simulink model "Kalman_EMPhase_noC"  (R2019b)
settings: Solver=FixedStepAuto  StartTime=0.0  StopTime=model.sim_dur  FixedStep=model.Ts  RelTol=1e-3
undefined symbols (not defined in the file or in its folder): Discrete, model, Time
libraries: dspsrcs4 x10, dspindex x4, ctrlSharedLib x2
settings Model: Creator=isidoraradenkovic  LastModifiedBy=isidoraradenkovic

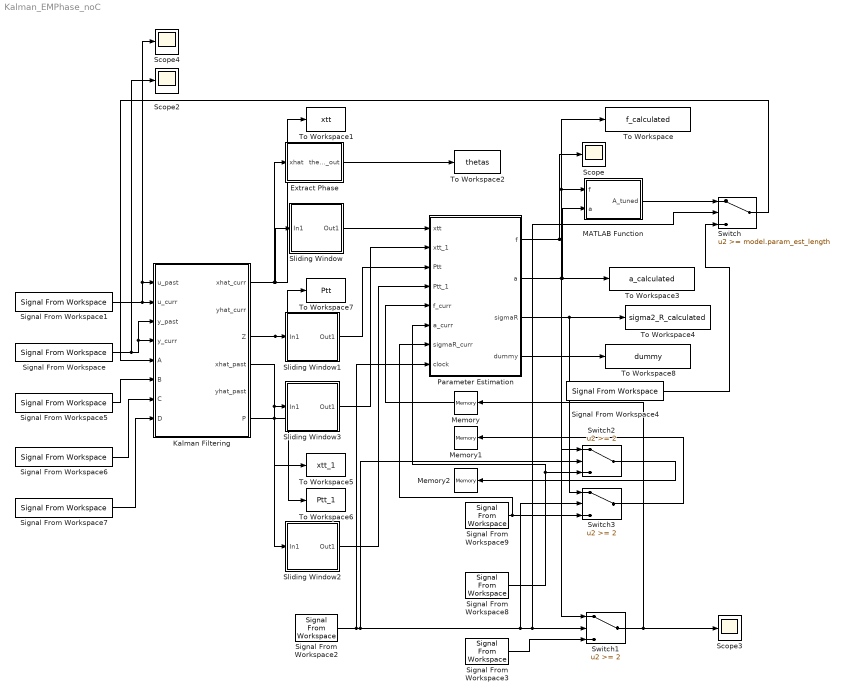
== system Kalman_EMPhase_noC ==
  Extract Phase : MATLAB Function  TreatAsAtomicUnit=on  SystemSampleTime=model.Ts
  Kalman Filtering : Subsystem
  MATLAB Function : MATLAB Function  TreatAsAtomicUnit=on  SystemSampleTime=model.Ts
  Memory : Memory
  Memory1 : Memory
  Memory2 : Memory
  Parameter Estimation : MATLAB Function  TreatAsAtomicUnit=on  SystemSampleTime=model.Ts
  Scope{,2..4} (4 alike) : Scope
  Signal From Workspace : dspsrcs4/Signal From Workspace  X=input_data  Ts=model.Ts  nsamps=1  OutputAfterFinalValue=Cyclic repetition  ignoreOrWarnInputAndFrameLengths=off  OutputFrames=off
  Signal From Workspace1 : dspsrcs4/Signal From Workspace  X=tms_pulses  Ts=model.Ts  nsamps=1  OutputAfterFinalValue=Cyclic repetition  ignoreOrWarnInputAndFrameLengths=off  OutputFrames=off
  Signal From Workspace2 : dspsrcs4/Signal From Workspace  X=1:1:(6*model.param_est_length)  Ts=model.Ts  nsamps=1  OutputAfterFinalValue=Holding final value  ignoreOrWarnInputAndFrameLengths=off  OutputFrames=off
  Signal From Workspace3 : dspsrcs4/Signal From Workspace  X=model.f  Ts=model.Ts  nsamps=1  OutputAfterFinalValue=Cyclic repetition  ignoreOrWarnInputAndFrameLengths=off  OutputFrames=off
  Signal From Workspace4 : dspsrcs4/Signal From Workspace  X=model.A  Ts=model.Ts/2  nsamps=2  OutputAfterFinalValue=Cyclic repetition  ignoreOrWarnInputAndFrameLengths=off  OutputFrames=off
  Signal From Workspace5 : dspsrcs4/Signal From Workspace  X=model.B  Ts=model.Ts/2  nsamps=2  OutputAfterFinalValue=Cyclic repetition  ignoreOrWarnInputAndFrameLengths=off  OutputFrames=off
  Signal From Workspace6 : dspsrcs4/Signal From Workspace  X=model.C  Ts=model.Ts  nsamps=1  OutputAfterFinalValue=Cyclic repetition  ignoreOrWarnInputAndFrameLengths=off  OutputFrames=off
  Signal From Workspace7 : dspsrcs4/Signal From Workspace  X=model.D  Ts=model.Ts  nsamps=1  OutputAfterFinalValue=Cyclic repetition  ignoreOrWarnInputAndFrameLengths=off  OutputFrames=off
  Signal From Workspace8 : dspsrcs4/Signal From Workspace  X=model.a  Ts=model.Ts/2  nsamps=2  OutputAfterFinalValue=Cyclic repetition  ignoreOrWarnInputAndFrameLengths=off  OutputFrames=off
  Signal From Workspace9 : dspsrcs4/Signal From Workspace  X=model.sigma2_R  Ts=model.Ts  nsamps=1  OutputAfterFinalValue=Cyclic repetition  ignoreOrWarnInputAndFrameLengths=off  OutputFrames=off
  Sliding Window : Subsystem
  Sliding Window1 : Subsystem
  Sliding Window2 : Subsystem
  Sliding Window3 : Subsystem
  Switch : Switch  Threshold=model.param_est_length
  Switch1 : Switch  Threshold=2
  Switch2 : Switch  Threshold=2
  Switch3 : Switch  Threshold=2
  To Workspace : ToWorkspace  VariableName=f_calculated  SampleTime=model.Ts
      settings: MaxDataPoints=1  Save2DSignal=2-D array (concatenate along first dimension)
  To Workspace1 : ToWorkspace  VariableName=xtt  SampleTime=model.Ts
      settings: Save2DSignal=2-D array (concatenate along first dimension)
  To Workspace2 : ToWorkspace  VariableName=thetas  SampleTime=model.Ts
      settings: Save2DSignal=2-D array (concatenate along first dimension)
  To Workspace3 : ToWorkspace  VariableName=a_calculated  SampleTime=model.Ts
      settings: MaxDataPoints=2  Save2DSignal=2-D array (concatenate along first dimension)
  To Workspace4 : ToWorkspace  VariableName=sigma2_R_calculated  SampleTime=model.Ts
      settings: MaxDataPoints=1  Save2DSignal=2-D array (concatenate along first dimension)
  To Workspace5 : ToWorkspace  VariableName=xtt_1  SampleTime=model.Ts
      settings: Save2DSignal=2-D array (concatenate along first dimension)
  To Workspace6 : ToWorkspace  VariableName=Ptt_1  SampleTime=model.Ts
      settings: Save2DSignal=2-D array (concatenate along first dimension)
  To Workspace7 : ToWorkspace  VariableName=Ptt  SampleTime=model.Ts
      settings: Save2DSignal=2-D array (concatenate along first dimension)
  To Workspace8 : ToWorkspace  VariableName=dummy  SampleTime=model.Ts
      settings: Save2DSignal=2-D array (concatenate along first dimension)
  wires:
  Signal From Workspace/1 -> Kalman Filtering/3(y_past), Kalman Filtering/4(y_curr), Scope2/1
  Parameter Estimation/1(f) -> To Workspace/1, MATLAB Function/1(f), Switch1/1, Scope/1
  Signal From Workspace2/1 -> Switch/2, Switch1/2, Switch3/2, Switch2/2, Parameter Estimation/8(clock)
  Switch1/1 -> Scope3/1, Memory/1
  Parameter Estimation/3(sigmaR) -> Switch3/1, To Workspace4/1
  Switch3/1 -> Memory1/1
  Kalman Filtering/6(P) -> To Workspace6/1, Sliding Window2/1(In1)
  Kalman Filtering/1(xhat_curr) -> Sliding Window/1(In1), To Workspace1/1, Extract Phase/1(xhat)
  Signal From Workspace1/1 -> Kalman Filtering/1(u_past), Scope4/1, Kalman Filtering/2(u_curr)
  Sliding Window/1(Out1) -> Parameter Estimation/1(xtt)
  Signal From Workspace4/1 -> Switch/3
  MATLAB Function/1(A_tuned) -> Switch/1
  Extract Phase/1(thetas_out) -> To Workspace2/1
  Sliding Window2/1(Out1) -> Parameter Estimation/4(Ptt_1)
  Switch2/1 -> Memory2/1
  Parameter Estimation/2(a) -> To Workspace3/1, MATLAB Function/2(a), Switch2/1
  Sliding Window1/1(Out1) -> Parameter Estimation/3(Ptt)
  Signal From Workspace3/1 -> Switch1/3
  Kalman Filtering/3(Z) -> Sliding Window1/1(In1), To Workspace7/1
  Signal From Workspace5/1 -> Kalman Filtering/6(B)
  Kalman Filtering/4(xhat_past) -> Sliding Window3/1(In1), To Workspace5/1
  Switch/1 -> Kalman Filtering/5(A)
  Signal From Workspace6/1 -> Kalman Filtering/7(C)
  Signal From Workspace9/1 -> Parameter Estimation/7(sigmaR_curr), Switch3/3
  Signal From Workspace7/1 -> Kalman Filtering/8(D)
  Signal From Workspace8/1 -> Parameter Estimation/6(a_curr), Switch2/3
  Parameter Estimation/4(dummy) -> To Workspace8/1
  Sliding Window3/1(Out1) -> Parameter Estimation/2(xtt_1)
  Memory/1 -> Parameter Estimation/5(f_curr)

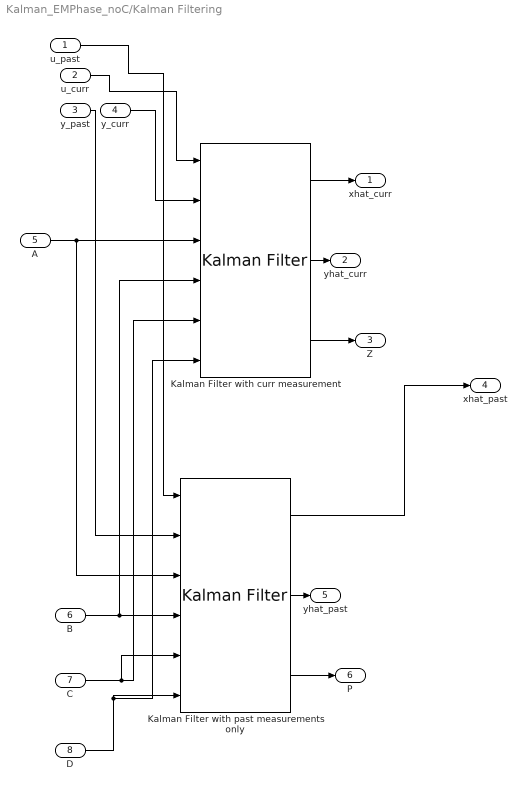
== system Kalman_EMPhase_noC/Kalman Filtering ==
  u_past : Inport
  u_curr : Inport  Port=2
  y_past : Inport  Port=3
  y_curr : Inport  Port=4
  A : Inport  Port=5
  B : Inport  Port=6
  C : Inport  Port=7
  D : Inport  Port=8
  Kalman Filter with curr measurement : ctrlSharedLib/Kalman Filter  TimeDomain=Discrete-Time  UseCurrentEstimator=on  ModelSource=Input port  ModelSourceVariable=ss(0.95,1,1,0,1)  A=model.A  B=model.B  C=model.C  D=0  NumberOfStates=2  NumberOfInputs=1  NumberOfOutputs=1  InitialEstimateSource=Dialog  X0=model.x_0  P0=model.Q_const  UseK=off  UseGH=on  NumberOfProcessNoiseInputs=1  G=model.Gm  TimeInvariantG=on  H=0  TimeInvariantH=on  Q=model.Q  TimeInvariantQ=on  R=model.R  TimeInvariantR=on  N=0  TimeInvariantN=on  AddInputPort=on  AddEnablePort=off  OutputEstimatedY=on  OutputP=on  Ts=model.Ts
      settings: SourceProductBaseCode=CT
  Kalman Filter with past measurements only : ctrlSharedLib/Kalman Filter  TimeDomain=Discrete-Time  UseCurrentEstimator=off  ModelSource=Input port  ModelSourceVariable=ss(0.95,1,1,0,1)  A=model.A  B=model.B  C=model.C  D=0  NumberOfStates=2  NumberOfInputs=1  NumberOfOutputs=1  InitialEstimateSource=Dialog  X0=model.x_0  P0=model.Q_const  UseK=off  UseGH=on  NumberOfProcessNoiseInputs=1  G=model.Gm  TimeInvariantG=on  H=0  TimeInvariantH=on  Q=model.Q  TimeInvariantQ=on  R=model.R  TimeInvariantR=on  N=0  TimeInvariantN=on  AddInputPort=on  AddEnablePort=off  OutputEstimatedY=on  OutputP=on  Ts=model.Ts
      settings: SourceProductBaseCode=CT
  xhat_curr : Outport
  yhat_curr : Outport  Port=2
  Z : Outport  Port=3
  xhat_past : Outport  Port=4
  yhat_past : Outport  Port=5
  P : Outport  Port=6
  wires:
  Kalman Filter with past measurements only/2 -> yhat_past/1
  A/1 -> Kalman Filter with past measurements only/3, Kalman Filter with curr measurement/3
  Kalman Filter with curr measurement/2 -> yhat_curr/1
  y_past/1 -> Kalman Filter with past measurements only/2
  Kalman Filter with past measurements only/3 -> P/1
  D/1 -> Kalman Filter with curr measurement/6, Kalman Filter with past measurements only/6
  u_curr/1 -> Kalman Filter with curr measurement/1
  Kalman Filter with curr measurement/1 -> xhat_curr/1
  C/1 -> Kalman Filter with curr measurement/5, Kalman Filter with past measurements only/5
  u_past/1 -> Kalman Filter with past measurements only/1
  y_curr/1 -> Kalman Filter with curr measurement/2
  Kalman Filter with past measurements only/1 -> xhat_past/1
  Kalman Filter with curr measurement/3 -> Z/1
  B/1 -> Kalman Filter with curr measurement/4, Kalman Filter with past measurements only/4

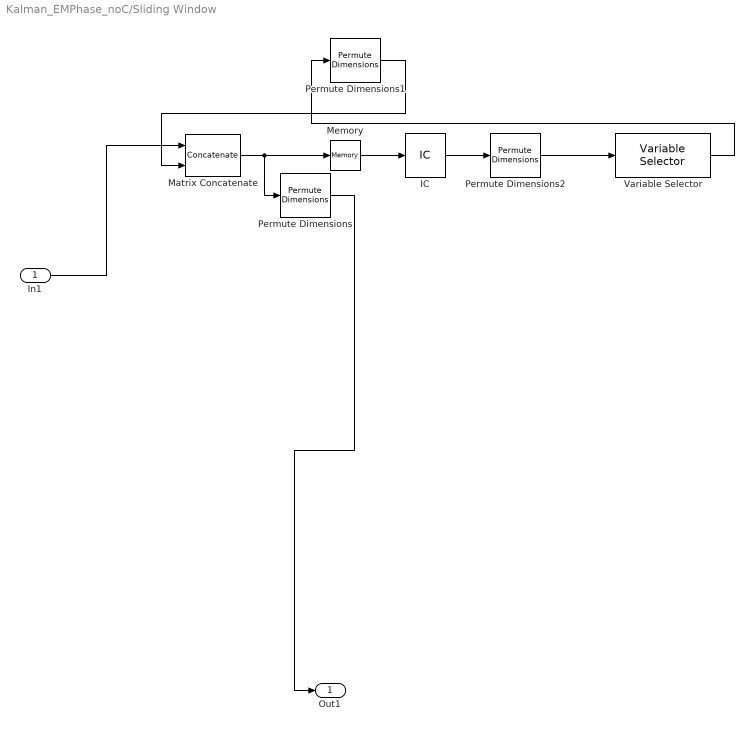
== system Kalman_EMPhase_noC/Sliding Window ==
  In1 : Inport
  IC : InitialCondition  Value=zeros(2, model.param_est_length+1)
  Matrix Concatenate : Concatenate  Mode=Multidimensional array  ConcatenateDimension=2
  Memory : Memory  InheritSampleTime=on
  Permute Dimensions : PermuteDimensions
  Permute Dimensions1 : PermuteDimensions
  Permute Dimensions2 : PermuteDimensions
  Variable Selector : dspindex/Variable Selector  NumInputs=1  rowsOrCols=Rows  IdxMode=Fixed  Elements=2:(model.param_est_length+1)  ZerOneIdxMode=One-based  errmode=Clip Index  FillMode=on  FillValues=0
  Out1 : Outport
  wires:
  In1/1 -> Matrix Concatenate/1
  Permute Dimensions/1 -> Out1/1
  Permute Dimensions2/1 -> Variable Selector/1
  IC/1 -> Permute Dimensions2/1
  Variable Selector/1 -> Permute Dimensions1/1
  Memory/1 -> IC/1
  Permute Dimensions1/1 -> Matrix Concatenate/2
  Matrix Concatenate/1 -> Permute Dimensions/1, Memory/1

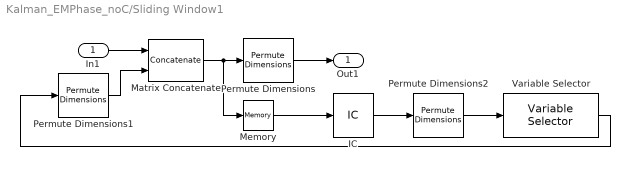
== system Kalman_EMPhase_noC/Sliding Window1 ==
  In1 : Inport
  IC : InitialCondition  Value=zeros(2, 2*(model.param_est_length+1))
  Matrix Concatenate : Concatenate  Mode=Multidimensional array  ConcatenateDimension=2
  Memory : Memory  InheritSampleTime=on
  Permute Dimensions : PermuteDimensions
  Permute Dimensions1 : PermuteDimensions
  Permute Dimensions2 : PermuteDimensions
  Variable Selector : dspindex/Variable Selector  NumInputs=1  rowsOrCols=Rows  IdxMode=Fixed  Elements=3:2*(model.param_est_length+1)  ZerOneIdxMode=One-based  errmode=Clip Index  FillMode=on  FillValues=0
  Out1 : Outport
  wires:
  In1/1 -> Matrix Concatenate/1
  Matrix Concatenate/1 -> Permute Dimensions/1, Memory/1
  Permute Dimensions/1 -> Out1/1
  Permute Dimensions2/1 -> Variable Selector/1
  IC/1 -> Permute Dimensions2/1
  Variable Selector/1 -> Permute Dimensions1/1
  Memory/1 -> IC/1
  Permute Dimensions1/1 -> Matrix Concatenate/2

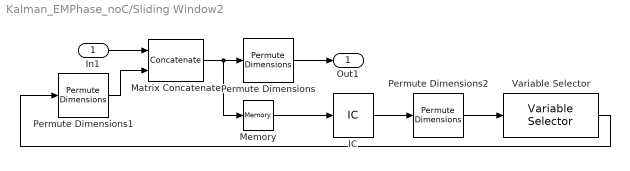
== system Kalman_EMPhase_noC/Sliding Window2 ==
  In1 : Inport
  IC : InitialCondition  Value=zeros(2, 2*(model.param_est_length+1))
  Matrix Concatenate : Concatenate  Mode=Multidimensional array  ConcatenateDimension=2
  Memory : Memory  InheritSampleTime=on
  Permute Dimensions : PermuteDimensions
  Permute Dimensions1 : PermuteDimensions
  Permute Dimensions2 : PermuteDimensions
  Variable Selector : dspindex/Variable Selector  NumInputs=1  rowsOrCols=Rows  IdxMode=Fixed  Elements=3:2*(model.param_est_length+1)  ZerOneIdxMode=One-based  errmode=Clip Index  FillMode=on  FillValues=0
  Out1 : Outport
  wires:
  In1/1 -> Matrix Concatenate/1
  Matrix Concatenate/1 -> Permute Dimensions/1, Memory/1
  Permute Dimensions/1 -> Out1/1
  Permute Dimensions2/1 -> Variable Selector/1
  IC/1 -> Permute Dimensions2/1
  Variable Selector/1 -> Permute Dimensions1/1
  Memory/1 -> IC/1
  Permute Dimensions1/1 -> Matrix Concatenate/2

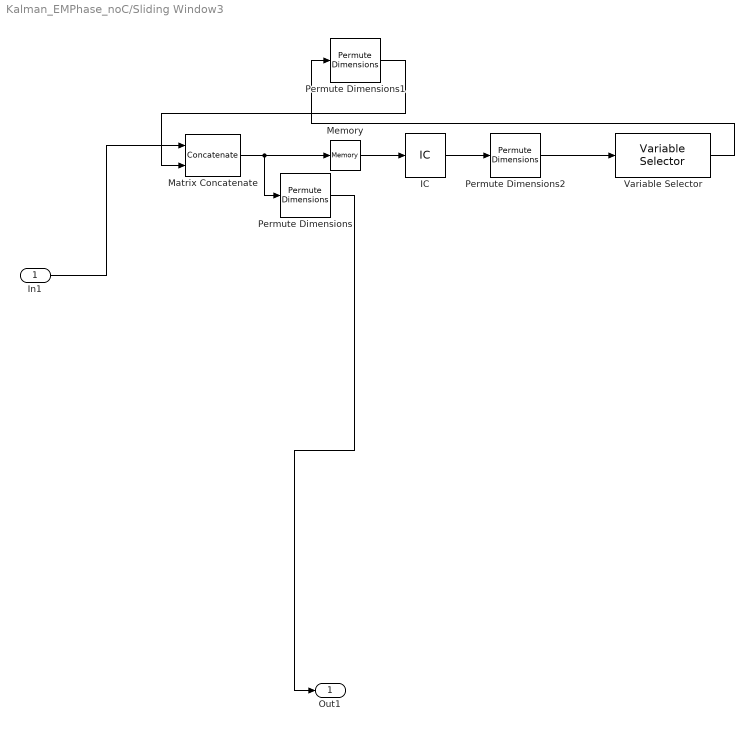
== system Kalman_EMPhase_noC/Sliding Window3 ==
  In1 : Inport
  IC : InitialCondition  Value=zeros(2, model.param_est_length+1)
  Matrix Concatenate : Concatenate  Mode=Multidimensional array  ConcatenateDimension=2
  Memory : Memory  InheritSampleTime=on
  Permute Dimensions : PermuteDimensions
  Permute Dimensions1 : PermuteDimensions
  Permute Dimensions2 : PermuteDimensions
  Variable Selector : dspindex/Variable Selector  NumInputs=1  rowsOrCols=Rows  IdxMode=Fixed  Elements=2:(model.param_est_length+1)  ZerOneIdxMode=One-based  errmode=Clip Index  FillMode=on  FillValues=0
  Out1 : Outport
  wires:
  In1/1 -> Matrix Concatenate/1
  Permute Dimensions/1 -> Out1/1
  Permute Dimensions2/1 -> Variable Selector/1
  IC/1 -> Permute Dimensions2/1
  Variable Selector/1 -> Permute Dimensions1/1
  Memory/1 -> IC/1
  Permute Dimensions1/1 -> Matrix Concatenate/2
  Matrix Concatenate/1 -> Permute Dimensions/1, Memory/1

== matlab function Kalman_EMPhase_noC/Parameter Estimation ==
  settings: sampleTime=1
  data: xtt input; xtt_1 input; Ptt input; f output size=model.num_rhythms; Ptt_1 input; a output size=[2*model.num_rhythms, 2*model.num_rhythms]; sigmaR output size=model.num_rhythms; model parameter; f_curr input; a_curr input; sigmaR_curr input; clock input; dummy output
function [f, a, sigmaR, dummy]  = parameter_estimation(xtt, xtt_1, Ptt, Ptt_1, model, f_curr, a_curr, sigmaR_curr, clock)

%WARNING!!!!!! To-do: add dimensions_param = model.state_dimensions;
%Right now, 2 is used as a dimension because Simulink complains when
%variables are used for matrix dimensions. When the state space is
%extended for artefact removal, change the 2's to a new value.
%Warning No2: note the limits imposed on model parameters, such as how
%many samples we use to do EM. If this starts causing errors, ensure
%that you are using last n samples where n is at most the max used here.
%model = model;

f = f_curr;
a = a_curr;
sigmaR = sigmaR_curr;
dummy = [1 2; 3 4];

if clock == model.param_est_length+2 %&& clock <= model.param_est_length+5
    %%Backward Smoothing
    [PttN, xttN, Ptt_1N, xforwN, PforwN] = backward_smoothing(model, Ptt, Ptt_1, xtt, xtt_1);
    
    %%EM parameter estimation
    [f, a, sigmaR, dummy]  = em_method(model, PttN, xttN, Ptt_1N, xforwN, PforwN);
    
end

    function [PttN, xttN, Ptt_1N, xNfinal, PNfinal] = backward_smoothing(model, Ptt, Ptt_1, xtt, xtt_1)
        length_param = model.param_est_length; %Limit to a max of 5000, BUT product limit is 10000
        
        PttN = zeros(min(2 * length_param, 10000), 2); % For the smoothing step
        xttN = zeros(min(length_param, 5000), 2);
        Ptt_1N = zeros(min(2 * length_param, 10000), 2); % Covariance
        
        xforwN = xtt(length_param+1, :);
        PforwN = Ptt((2 * length_param+1):(2 * (length_param+1)), :);
        
        xNfinal = xforwN;
        PNfinal = PforwN;
        
        for j= (length_param+1):(-1):2 % The paper is 0 indexed, MATLAB is 1 indexed
            % Extract matrices for simpler representation
            % Index (j-1) becomes:
            % ((j-2)*dimensions_param+1):((j-1)*dimensions_param)
            % Index j becomes:
            % ((j-1)*dimensions_param+1):(j*dimensions_param)
            
            ind_prev = max((j-2)*2+1, 1):min((j-1)*2, 50000);
            ind_curr = max((j-1)*2+1, 1):min(j*2, 50000);
            
            Pt_1_prev = Ptt_1(ind_prev, :);
            Pt_1_curr = Ptt_1(ind_curr, :);
            %Pt_prev = Ptt(ind_prev, :);
            xt_prev = xtt_1(j-1, 1:2);
            
            J = Pt_1_prev*model.A'*pinv(Pt_1_curr);
            xttN(j-1, min(1:2, 10:11)) = xt_prev+(xforwN-xt_prev*(model.A'))*(J');
            PttN(ind_prev, min(1:2, 10:11)) = Pt_1_prev+J*(PforwN-Pt_1_curr)*J';
            %covariance is symmetric, so Ptt_1N = Pt_1tN = J*PttN hence:
            Ptt_1N(ind_prev, min(1:2, 10:11)) = J*PforwN;
            
            xforwN = xttN(j-1, :);
            PforwN = PttN(ind_prev, :);
        end
        
    end

    function [f, a, sigmaR, dummy]  = em_method(model, PttN, xttN, Ptt_1N, xNfinal, PNfinal)
        length_param = model.param_est_length;
        num_rhythms = model.num_rhythms;
        
        P_A = matrix_sum(PttN, 2);
        P_B = matrix_sum(Ptt_1N, 2);
        P_C = matrix_sum([PttN((2+1):end, :); PNfinal], 2);
        
        xtN = [xttN(2:min(length_param, 5000), :); xNfinal];
        x_A_prod = matrix_product(xttN, xttN, 2);
        x_A = matrix_sum(x_A_prod, 2);
        x_B_prod = matrix_product(xtN, xttN, 2);
        x_B = matrix_sum(x_B_prod, 2);
        x_C_prod = matrix_product(xtN, xtN, 2);
        x_C = matrix_sum(x_C_prod, 2);
        
        A_smooth = P_A+x_A;
        B_smooth = P_B+x_B;
        C_smooth = P_C+x_C;
        
        denum_temp = tr(B_smooth, num_rhythms);
        denum = denum_temp(1);
        f_temp = 0.5*pi;
        if denum ~= 0
            f_temp = atan(double(rt(B_smooth, num_rhythms))./double(tr(B_smooth, num_rhythms)));
        end
        
        a_temp = sqrt(rt(B_smooth, num_rhythms).^2+tr(B_smooth, num_rhythms).^2)./tr(A_smooth, num_rhythms);
        sigmaR_temp = double(tr(C_smooth, num_rhythms)-(a_temp.^2).*tr(A_smooth, num_rhythms))./double(2*length_param);
        
        %f_temp2 = mod(double(f_temp(1)/pi+50000), 2)*pi;
        f = f_temp(1);
        %f = length(f_temp);
        a = a_temp(1)*eye(2);
        sigmaR = sigmaR_temp(1);
        dummy = P_A;
    end

end

== matlab function Kalman_EMPhase_noC/Extract Phase ==
  settings: updateMethod=DISCRETE  sampleTime=model.Ts
  data: xhat input; thetas_out output
function thetas_out  = extract_phase(xhat)
num_rhythms = length(xhat)/2;
% thetas_out = zeros(num_rhythms, 1);
% 
% for j = 1:num_rhythms
%     Im = xhat(2 * (j-1) + 2);
%     Re = xhat(2 * (j-1) + 1);
%     thetas_out(j, 1) = atan2(Im, Re);
% end

thetas_out = atan2(xhat(2:2:2*num_rhythms), xhat(1:2:2*(num_rhythms-1)+1))

== matlab function Kalman_EMPhase_noC/MATLAB Function ==
  data: A_tuned output; f input; a input; model parameter
function A_tuned = tune_A(f, a, model)
angles = 2*pi*model.Ts*f;
rot_cell = cell(1); % GENERALISE FOR MULTIPLE FREQ TRACKING

for j = 1:1 % model.num_rhythms GENERALISE FOR MULTIPLE FREQ TRACKING
    rot_j = [cos(angles(j)) -sin(angles(j)); sin(angles(j)) cos(angles(j))];
    rot_cell{j} = rot_j;
end
rot =blkdiag(rot_cell{1}); % GENERALISE FOR MULTIPLE FREQ TRACKING

A_tuned = a*rot;
